simulink model "sampleModel69"  (Simulink 9.1)
settings: Solver=VariableStepAuto  StartTime=0.0  StopTime=10.0  RelTol=1e-3
undefined symbols (not defined in the file): DiscIntNeverNeededParam, Newton, Raphson
libraries: simulink x28
settings Model: SuppressorTable="22 serialization::archive 11 0 6 0 0 1 8 0 0 0 0 6 0 0 1 0 21 sampleModel69/cfblk24 0 6 0 0 2 8 0 0 0 0 6 41 Simulink:DataType:WarningOverFlowDetected 0 0 0 6 0  0  0 0 0 0 8 20160523 0 0 0 10 57 55 0 1 40 SimulinkFixedPoint:util:Overflowoccurred 0 0 0  0  8 20160523 0 10 57 55 0 1"  Creator=DELL  LastModifiedBy=DELL
settings DataIOCC: SaveFormat=Dataset
settings OptimizationCC: LifeSpan=auto
settings DebuggingCC: UnderspecifiedInitializationDetection=Simplified  MergeDetectMultiDrivingBlocksExec=error  SFUnexpectedBacktrackingDiag=error  SFNoUnconditionalDefaultTransitionDiag=error  SFExecutionAtInitializationDiag=warning
settings HardwareCC: ProdBitPerPointer=64  ProdBitPerSizeT=64  ProdBitPerPtrDiffT=64  ProdLargestAtomicFloat=Float  ProdIntDivRoundTo=Zero  ProdEndianess=LittleEndian  ProdWordSize=64  ProdHWDeviceType=Intel->x86-64 (Windows64)
settings ModelReferenceCC: PropagateSignalLabelsOutOfModel=on
settings CodeAppCC: StateflowObjectComments=off
settings GRTTargetCC: TargetLangStandard=C99 (ISO)  CombineOutputUpdateFcns=on  GRTInterface=off
settings ConfigComp: CovMetricSettings=dwe  CovHtmlReporting=off  CovSaveCumulativeToWorkspaceVar=off  CovSaveSingleToWorkspaceVar=off  CovExternalEMLEnable=on

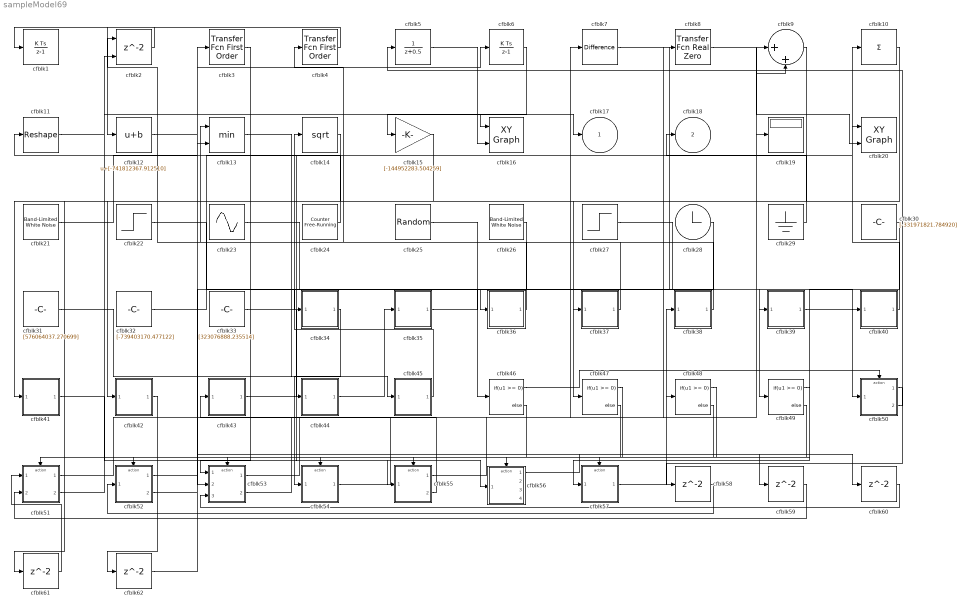
== system sampleModel69 ==
  cfblk1 : DiscreteIntegrator  ICPrevOutput=DiscIntNeverNeededParam  ICPrevScaledInput=DiscIntNeverNeededParam
  cfblk10 : Sum  Inputs=+
  cfblk11 : Reshape
  cfblk12 : Bias  Bias=[-741812367.912510]
  cfblk13 : MinMax  Inputs=2
  cfblk14 : Sqrt  SaturateOnIntegerOverflow=on
  cfblk15 : Gain  Gain=[-144952283.504259]
  cfblk16 : simulink/Sinks/XY Graph  xmin=-1  xmax=1  ymin=-1  ymax=1  st=-1
  cfblk19 : Display
  cfblk2 : Delay  ShowEnablePort=on  SampleTime=1
      settings: InputPortMap=u0,e6
  cfblk20 : simulink/Sinks/XY Graph  xmin=-1  xmax=1  ymin=-1  ymax=1  st=-1
  cfblk21 : simulink/Sources/Band-Limited White Noise  Cov=[6037447037.937979]  Ts=0.1  seed=[876082566.000000]
  cfblk22 : Step  Time=[11.000000]  Before=[-275297189.840630]  After=[-539641405.441389]  SampleTime=0
  cfblk23 : Sin  Amplitude=[-719520156.882693]  Bias=[435795628.391906]  SampleTime=0
  cfblk24 : simulink/Sources/Counter Free-Running  NumBits=[17.000000]  tsamp=-1
  cfblk25 : RandomNumber  Mean=[13472.399108]  Variance=[10146.259517]  Seed=[945900155.000000]  SampleTime=0.1
  cfblk26 : simulink/Sources/Band-Limited White Noise  Cov=[3648562607.707092]  Ts=0.1  seed=[6350696125.000000]
  cfblk27 : Step  Time=[48.000000]  Before=[68635987.034339]  After=[-934709305.033642]  SampleTime=0
  cfblk28 : Clock
  cfblk29 : Ground
  cfblk3 : simulink/Discrete/Transfer Fcn First Order  PoleZ=0.95  ICPrevOutput=0.0  DoSatur=off
      settings: SourceProductName=Simulink
  cfblk30 : Constant  Value=[-331971821.784920]  SampleTime=1
  cfblk31 : Constant  Value=[576064037.270699]  SampleTime=1
  cfblk32 : Constant  Value=[-739403170.477122]  SampleTime=1
  cfblk33 : Constant  Value=[323076888.235514]  SampleTime=1
  cfblk34 : Subsystem
  cfblk35 : Subsystem
  cfblk36 : Subsystem
  cfblk37 : Subsystem
  cfblk38 : Subsystem
  cfblk39 : Subsystem
  cfblk4 : simulink/Discrete/Transfer Fcn First Order  PoleZ=0.95  ICPrevOutput=0.0  DoSatur=off
      settings: SourceProductName=Simulink
  cfblk40 : Subsystem
  cfblk41 : Subsystem
  cfblk42 : Subsystem
  cfblk43 : Subsystem
  cfblk44 : Subsystem
  cfblk45 : Subsystem
  cfblk{46..49} (4 alike) : If  IfExpression=u1 >= 0  SampleTime=1
  cfblk5 : DiscreteTransferFcn  SampleTime=1
  cfblk50 : Subsystem  TreatAsAtomicUnit=on
  cfblk51 : Subsystem  TreatAsAtomicUnit=on
  cfblk52 : Subsystem  TreatAsAtomicUnit=on
  cfblk53 : Subsystem  TreatAsAtomicUnit=on
  cfblk54 : Subsystem  TreatAsAtomicUnit=on
  cfblk55 : Subsystem  TreatAsAtomicUnit=on
  cfblk56 : Subsystem  TreatAsAtomicUnit=on
  cfblk57 : Subsystem  TreatAsAtomicUnit=on
  cfblk{58..62} (5 alike) : Delay  SampleTime=1
  cfblk6 : DiscreteIntegrator  ICPrevOutput=DiscIntNeverNeededParam  ICPrevScaledInput=DiscIntNeverNeededParam
  cfblk7 : simulink/Discrete/Difference  ICPrevInput=0.0  OutMin=[]  OutMax=[]  OutDataTypeStr=Inherit: Inherit via back propagation  OutDataType=fixdt(1, 16)  OutScaling=2^-10  DoSatur=off
  cfblk8 : simulink/Discrete/Transfer Fcn Real Zero  ZeroZ=0.75  ICPrevInput=0.0  DoSatur=off
      settings: SourceProductName=Simulink  SourceProductBaseCode=SL
  cfblk9 : Sum  Inputs=|++
  cfblk17 : Outport
  cfblk18 : Outport  Port=2
  wires:
  cfblk34/1(cfblk2) -> cfblk54/1(cfblk1)
  cfblk23/1 -> cfblk47/1
  cfblk45/1(cfblk2) -> cfblk14/1
  cfblk22/1 -> cfblk36/1(cfblk1)
  cfblk9/1 -> cfblk41/1(cfblk1)
  cfblk13/1 -> cfblk45/1(cfblk1)
  cfblk32/1 -> cfblk10/1
  cfblk27/1 -> cfblk49/1
  cfblk7/1 -> cfblk39/1(cfblk1)
  cfblk14/1 -> cfblk42/1(cfblk1)
  cfblk30/1 -> cfblk57/1(cfblk1)
  cfblk38/1(cfblk2) -> cfblk13/1
  cfblk57/1(cfblk2) -> cfblk38/1(cfblk1)
  cfblk54/1(cfblk2) -> cfblk7/1
  cfblk24/1 -> cfblk11/1
  cfblk53/1(cfblk2) -> cfblk19/1
  cfblk40/1(cfblk2) -> cfblk20/1
  cfblk37/1(cfblk2) -> cfblk4/1
  cfblk4/1 -> cfblk12/1
  cfblk39/1(cfblk2) -> cfblk50/1(cfblk1)
  cfblk50/2(cfblk13) -> cfblk5/1
  cfblk12/1 -> cfblk16/1
  cfblk53/2(cfblk11) -> cfblk48/1
  cfblk51/1(cfblk2) -> cfblk9/1
  cfblk36/1(cfblk2) -> cfblk2/1
  cfblk3/1 -> cfblk53/1(cfblk1)
  cfblk33/1 -> cfblk55/1(cfblk1)
  cfblk2/1 -> cfblk1/1
  cfblk52/2(cfblk16) -> cfblk6/1
  cfblk8/1 -> cfblk20/2
  cfblk21/1 -> cfblk3/1
  cfblk55/1(cfblk2) -> cfblk8/1
  cfblk25/1 -> cfblk46/1
  cfblk43/1(cfblk2) -> cfblk9/2
  cfblk5/1 -> cfblk16/2
  cfblk29/1 -> cfblk18/1
  cfblk44/1(cfblk2) -> cfblk35/1(cfblk1)
  cfblk41/1(cfblk2) -> cfblk56/1(cfblk1)
  cfblk55/2(cfblk12) -> cfblk43/1(cfblk1)
  cfblk51/2(cfblk7) -> cfblk2/2
  cfblk28/1 -> cfblk34/1(cfblk1)
  cfblk10/1 -> cfblk37/1(cfblk1)
  cfblk35/1(cfblk2) -> cfblk40/1(cfblk1)
  cfblk31/1 -> cfblk44/1(cfblk1)
  cfblk26/1 -> cfblk53/2(cfblk9)
  cfblk11/1 -> cfblk17/1
  cfblk6/1 -> cfblk15/1
  cfblk46/1 -> cfblk50/Action
  cfblk46/2 -> cfblk51/Action
  cfblk47/1 -> cfblk52/Action
  cfblk47/2 -> cfblk53/Action
  cfblk48/1 -> cfblk54/Action
  cfblk48/2 -> cfblk55/Action
  cfblk49/1 -> cfblk56/Action
  cfblk49/2 -> cfblk57/Action
  cfblk50/1(cfblk2) -> cfblk58/1
  cfblk58/1 -> cfblk52/1(cfblk1)
  cfblk52/1(cfblk2) -> cfblk59/1
  cfblk59/1 -> cfblk51/2(cfblk6)
  cfblk56/1(cfblk2) -> cfblk60/1
  cfblk60/1 -> cfblk53/3(cfblk10)
  cfblk15/1 -> cfblk61/1
  cfblk61/1 -> cfblk51/1(cfblk1)
  cfblk42/1(cfblk2) -> cfblk62/1
  cfblk62/1 -> cfblk13/2

== system sampleModel69/cfblk34 ==
  cfblk1 : Inport
  cfblk2 : Outport
  wires:
  cfblk1/1 -> cfblk2/1

== system sampleModel69/cfblk35 ==
  cfblk1 : Inport
  cfblk2 : Outport
  wires:
  cfblk1/1 -> cfblk2/1

== system sampleModel69/cfblk36 ==
  cfblk1 : Inport
  cfblk2 : Outport
  wires:
  cfblk1/1 -> cfblk2/1

== system sampleModel69/cfblk37 ==
  cfblk1 : Inport
  cfblk2 : Outport
  wires:
  cfblk1/1 -> cfblk2/1

== system sampleModel69/cfblk38 ==
  cfblk1 : Inport
  cfblk2 : Outport
  wires:
  cfblk1/1 -> cfblk2/1

== system sampleModel69/cfblk39 ==
  cfblk1 : Inport
  cfblk2 : Outport
  wires:
  cfblk1/1 -> cfblk2/1

== system sampleModel69/cfblk40 ==
  cfblk1 : Inport
  cfblk2 : Outport
  wires:
  cfblk1/1 -> cfblk2/1

== system sampleModel69/cfblk41 ==
  cfblk1 : Inport
  cfblk2 : Outport
  wires:
  cfblk1/1 -> cfblk2/1

== system sampleModel69/cfblk42 ==
  cfblk1 : Inport
  cfblk2 : Outport
  wires:
  cfblk1/1 -> cfblk2/1

== system sampleModel69/cfblk43 ==
  cfblk1 : Inport
  cfblk2 : Outport
  wires:
  cfblk1/1 -> cfblk2/1

== system sampleModel69/cfblk44 ==
  cfblk1 : Inport
  cfblk2 : Outport
  wires:
  cfblk1/1 -> cfblk2/1

== system sampleModel69/cfblk45 ==
  cfblk1 : Inport
  cfblk2 : Outport
  wires:
  cfblk1/1 -> cfblk2/1

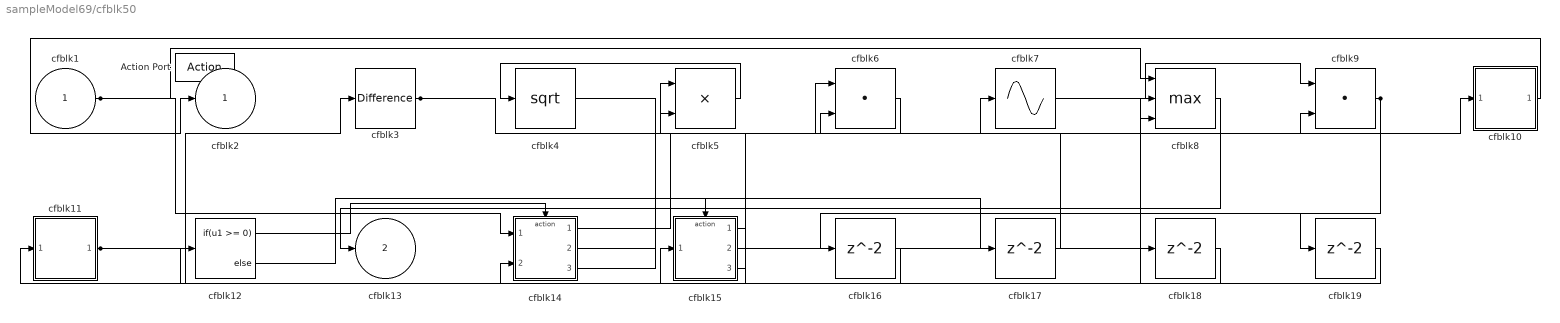
== system sampleModel69/cfblk50 ==
  cfblk1 : Inport
  Action Port : ActionPort  ActionType=then
  cfblk10 : Subsystem
  cfblk11 : Subsystem
  cfblk12 : If  IfExpression=u1 >= 0  SampleTime=1
  cfblk14 : Subsystem  TreatAsAtomicUnit=on
  cfblk15 : Subsystem  TreatAsAtomicUnit=on
  cfblk{16..19} (4 alike) : Delay
  cfblk3 : simulink/Discrete/Difference  ICPrevInput=0.0  OutMin=[]  OutMax=[]  OutDataTypeStr=Inherit: Inherit via back propagation  OutDataType=fixdt(1, 16)  OutScaling=2^-10  DoSatur=off
  cfblk4 : Sqrt  SaturateOnIntegerOverflow=on
  cfblk5 : Product  Inputs=**
  cfblk6 : DotProduct  InputSameDT=on  OutDataTypeStr=Inherit: Inherit via internal rule
  cfblk7 : Sin  TimeSource=Use external signal  SampleTime=0
  cfblk8 : MinMax  Function=max  Inputs=3
  cfblk9 : DotProduct  InputSameDT=on  OutDataTypeStr=Inherit: Inherit via internal rule
  cfblk2 : Outport
  cfblk13 : Outport  Port=2
  wires:
  cfblk8/1 -> cfblk13/1
  cfblk11/1(cfblk2) -> cfblk3/1, cfblk18/1
  cfblk5/1 -> cfblk4/1
  cfblk6/1 -> cfblk5/1
  cfblk15/1(cfblk2) -> cfblk11/1(cfblk1)
  cfblk14/1(cfblk2) -> cfblk10/1(cfblk1)
  cfblk3/1 -> cfblk6/2, cfblk8/3
  cfblk7/1 -> cfblk9/1
  cfblk1/1 -> cfblk8/1, cfblk14/1(cfblk1)
  cfblk9/1 -> cfblk16/1, cfblk19/1
  cfblk15/2(cfblk12) -> cfblk8/2
  cfblk14/2(cfblk8) -> cfblk7/1
  cfblk10/1(cfblk2) -> cfblk2/1
  cfblk15/3(cfblk13) -> cfblk5/2
  cfblk14/3(cfblk9) -> cfblk9/2
  cfblk12/1 -> cfblk14/Action
  cfblk12/2 -> cfblk15/Action
  cfblk16/1 -> cfblk15/1(cfblk1)
  cfblk4/1 -> cfblk17/1
  cfblk17/1 -> cfblk6/1
  cfblk18/1 -> cfblk12/1
  cfblk19/1 -> cfblk14/2(cfblk7)

== system sampleModel69/cfblk51 ==
  cfblk1 : Inport
  cfblk6 : Inport  Port=2
  Action Port : ActionPort  ActionType=else
  cfblk3 : DiscreteStateSpace  SampleTime=-1
  cfblk4 : simulink/Discrete/Transfer Fcn Real Zero  ZeroZ=0.75  ICPrevInput=0.0  DoSatur=off
      settings: SourceProductName=Simulink  SourceProductBaseCode=SL
  cfblk5 : Subsystem
  cfblk2 : Outport
  cfblk7 : Outport  Port=2
  wires:
  cfblk6/1 -> cfblk4/1
  cfblk1/1 -> cfblk5/1(cfblk1)
  cfblk4/1 -> cfblk7/1
  cfblk5/1(cfblk2) -> cfblk3/1
  cfblk3/1 -> cfblk2/1

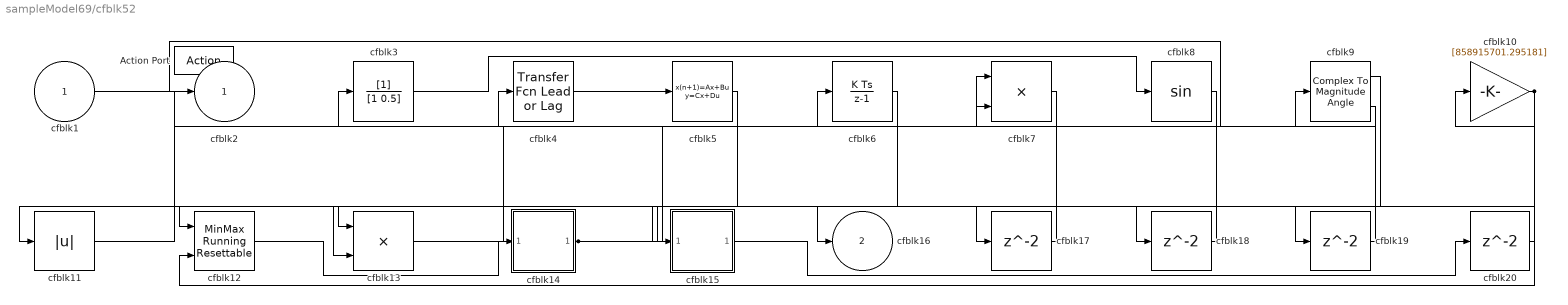
== system sampleModel69/cfblk52 ==
  cfblk1 : Inport
  Action Port : ActionPort  ActionType=then
  cfblk10 : Gain  Gain=[858915701.295181]
  cfblk11 : Abs
  cfblk12 : simulink/Math Operations/MinMax Running Resettable  Function=min  vinit=0.0
  cfblk13 : Product  Inputs=**
  cfblk14 : Subsystem
  cfblk15 : Subsystem
  cfblk{17..20} (4 alike) : Delay
  cfblk3 : DiscreteFilter
  cfblk4 : simulink/Discrete/Transfer Fcn Lead or Lag  PoleZ=0.95  ZeroZ=0.75  ICPrevOutput=0.0  ICPrevInput=0.0  DoSatur=off
      settings: SourceProductName=Simulink  SourceProductBaseCode=SL
  cfblk5 : DiscreteStateSpace  SampleTime=-1
  cfblk6 : DiscreteIntegrator  SampleTime=-1  ICPrevOutput=DiscIntNeverNeededParam  ICPrevScaledInput=DiscIntNeverNeededParam
  cfblk7 : Product  Inputs=**
  cfblk8 : Trigonometry
  cfblk9 : ComplexToMagnitudeAngle
  cfblk2 : Outport
  cfblk16 : Outport  Port=2
  wires:
  cfblk14/1(cfblk2) -> cfblk6/1, cfblk19/1
  cfblk3/1 -> cfblk8/1
  cfblk9/2 -> cfblk2/1
  cfblk4/1 -> cfblk5/1
  cfblk13/1 -> cfblk9/1
  cfblk5/1 -> cfblk12/1
  cfblk1/1 -> cfblk7/1
  cfblk7/1 -> cfblk13/2
  cfblk11/1 -> cfblk7/2
  cfblk10/1 -> cfblk12/2, cfblk16/1, cfblk15/1(cfblk1)
  cfblk12/1 -> cfblk14/1(cfblk1)
  cfblk6/1 -> cfblk11/1
  cfblk9/1 -> cfblk17/1
  cfblk17/1 -> cfblk13/1
  cfblk8/1 -> cfblk18/1
  cfblk18/1 -> cfblk3/1
  cfblk19/1 -> cfblk4/1
  cfblk15/1(cfblk2) -> cfblk20/1
  cfblk20/1 -> cfblk10/1

== system sampleModel69/cfblk53 ==
  cfblk1 : Inport
  cfblk9 : Inport  Port=2
  cfblk10 : Inport  Port=3
  Action Port : ActionPort  ActionType=else
  cfblk3 : simulink/Discrete/Difference  ICPrevInput=0.0  OutMin=[]  OutMax=[]  OutDataTypeStr=Inherit: Inherit via back propagation  OutDataType=fixdt(1, 16)  OutScaling=2^-10  DoSatur=off
  cfblk4 : DiscreteFilter
  cfblk5 : simulink/Math Operations/Slider Gain  gain=1  low=0  high=2
  cfblk6 : Sum  Inputs=+
  cfblk7 : Math  Operator=10^u  SaturateOnIntegerOverflow=on
  cfblk8 : Subsystem
  cfblk2 : Outport
  cfblk11 : Outport  Port=2
  wires:
  cfblk10/1 -> cfblk11/1
  cfblk3/1 -> cfblk7/1
  cfblk4/1 -> cfblk2/1
  cfblk9/1 -> cfblk6/1
  cfblk5/1 -> cfblk4/1
  cfblk1/1 -> cfblk3/1
  cfblk6/1 -> cfblk8/1(cfblk1)
  cfblk8/1(cfblk2) -> cfblk5/1

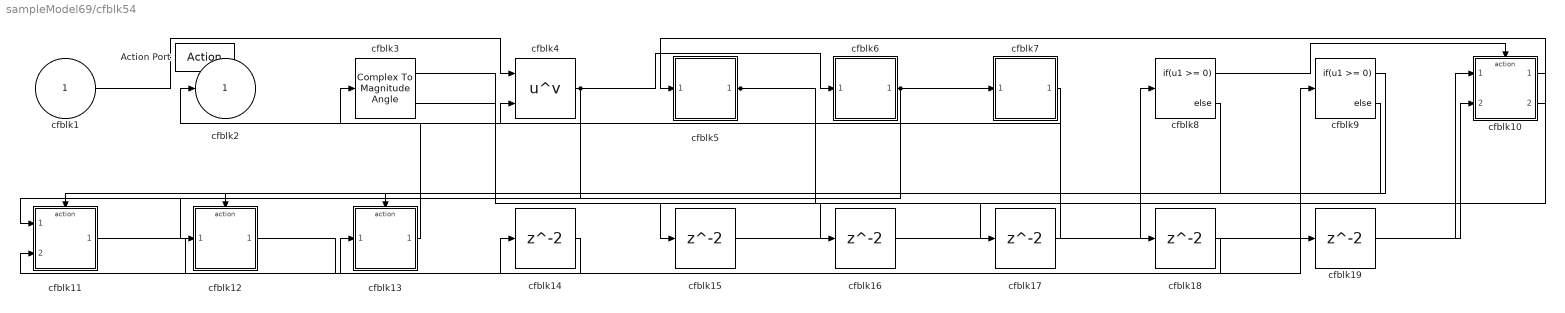
== system sampleModel69/cfblk54 ==
  cfblk1 : Inport
  Action Port : ActionPort  ActionType=then
  cfblk10 : Subsystem  TreatAsAtomicUnit=on
  cfblk11 : Subsystem  TreatAsAtomicUnit=on
  cfblk12 : Subsystem  TreatAsAtomicUnit=on
  cfblk13 : Subsystem  TreatAsAtomicUnit=on
  cfblk{14..19} (6 alike) : Delay
  cfblk3 : ComplexToMagnitudeAngle
  cfblk4 : Math  Operator=pow  SaturateOnIntegerOverflow=on
  cfblk5 : Subsystem
  cfblk6 : Subsystem
  cfblk7 : Subsystem
  cfblk8 : If  IfExpression=u1 >= 0  SampleTime=1
  cfblk9 : If  IfExpression=u1 >= 0  SampleTime=1
  cfblk2 : Outport
  wires:
  cfblk4/1 -> cfblk11/1(cfblk1), cfblk6/1(cfblk1)
  cfblk11/1(cfblk2) -> cfblk9/1
  cfblk13/1(cfblk2) -> cfblk3/1
  cfblk6/1(cfblk2) -> cfblk7/1(cfblk1), cfblk12/1(cfblk1)
  cfblk10/2(cfblk16) -> cfblk5/1(cfblk1)
  cfblk1/1 -> cfblk4/1
  cfblk5/1(cfblk2) -> cfblk17/1, cfblk18/1
  cfblk7/1(cfblk2) -> cfblk2/1
  cfblk8/1 -> cfblk10/Action
  cfblk8/2 -> cfblk11/Action
  cfblk9/1 -> cfblk12/Action
  cfblk9/2 -> cfblk13/Action
  cfblk12/1(cfblk2) -> cfblk14/1
  cfblk14/1 -> cfblk11/2(cfblk11)
  cfblk3/1 -> cfblk15/1
  cfblk15/1 -> cfblk10/1(cfblk1)
  cfblk10/1(cfblk2) -> cfblk16/1
  cfblk16/1 -> cfblk8/1
  cfblk17/1 -> cfblk4/2
  cfblk18/1 -> cfblk13/1(cfblk1)
  cfblk3/2 -> cfblk19/1
  cfblk19/1 -> cfblk10/2(cfblk15)

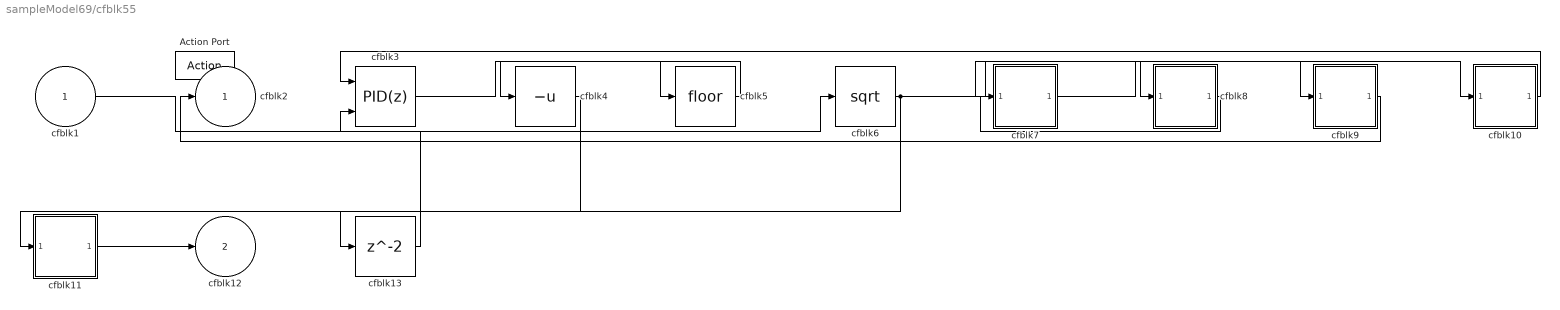
== system sampleModel69/cfblk55 ==
  cfblk1 : Inport
  Action Port : ActionPort  ActionType=else
  cfblk10 : Subsystem
  cfblk11 : Subsystem
  cfblk13 : Delay
  cfblk3 : simulink/Continuous/PID Controller (2DOF)  Controller=PID  TimeDomain=Discrete-time  SampleTime=-1  IntegratorMethod=Forward Euler  FilterMethod=Forward Euler  Form=Parallel  UseFilter=on  ControllerParametersSource=internal  P=1  I=1  D=0  N=100  b=1  c=1  InitialConditionSource=internal  InitialConditionForIntegrator=0  InitialConditionForFilter=0  ExternalReset=none  LimitOutput=off  UpperSaturationLimit=inf  LowerSaturationLimit=-inf  LinearizeAsGain=off  AntiWindupMode=none  Kb=1  TrackingMode=off  Kt=1  PParamMin=[]  PParamMax=[]  IParamMin=[]  IParamMax=[]  DParamMin=[]  DParamMax=[]  NParamMin=[]  NParamMax=[]  bParamMin=[]  bParamMax=[]  cParamMin=[]  cParamMax=[]  KbParamMin=[]  KbParamMax=[]  KtParamMin=[]  KtParamMax=[]  POutMin=[]  POutMax=[]  IOutMin=[]  IOutMax=[]  DOutMin=[]  DOutMax=[]  NOutMin=[]  NOutMax=[]  bOutMin=[]  bOutMax=[]  cOutMin=[]  cOutMax=[]  KbOutMin=[]  KbOutMax=[]  KtOutMin=[]  KtOutMax=[]  IntegratorOutMin=[]  IntegratorOutMax=[]  FilterOutMin=[]  FilterOutMax=[]  SumOutMin=[]  SumOutMax=[]  Sum1OutMin=[]  Sum1OutMax=[]  Sum2OutMin=[]  Sum2OutMax=[]  Sum3OutMin=[]  Sum3OutMax=[]  SumI1OutMin=[]  SumI1OutMax=[]  SumI2OutMin=[]  SumI2OutMax=[]  SumI3OutMin=[]  SumI3OutMax=[]  SumDOutMin=[]  SumDOutMax=[]  SaturationOutMin=[]  SaturationOutMax=[]  IntegratorContinuousStateAttributes=''  IntegratorStateMustResolveToSignalObject=off  IntegratorRTWStateStorageClass=Auto  FilterContinuousStateAttributes=''  FilterStateMustResolveToSignalObject=off  FilterRTWStateStorageClass=Auto  DifferentiatorICPrevScaledInput=0  DifferentiatorOutMin=[]  DifferentiatorOutMax=[]  FilterDiffOutCoefMin=[]  FilterDiffOutCoefMax=[]  SumDenOutMin=[]  SumDenOutMax=[]  SumNumOutMin=[]  SumNumOutMax=[]  ReciprocalOutMin=[]  ReciprocalOutMax=[]  DivideOutMin=[]  DivideOutMax=[]  TunerSelectOption=Transfer Function Based (PID Tuner App)
  cfblk4 : UnaryMinus
  cfblk5 : Rounding
  cfblk6 : Sqrt  SaturateOnIntegerOverflow=on
  cfblk7 : Subsystem
  cfblk8 : Subsystem
  cfblk9 : Subsystem
  cfblk2 : Outport
  cfblk12 : Outport  Port=2
  wires:
  cfblk6/1 -> cfblk8/1(cfblk1), cfblk11/1(cfblk1), cfblk10/1(cfblk1)
  cfblk8/1(cfblk2) -> cfblk7/1(cfblk1)
  cfblk10/1(cfblk2) -> cfblk3/1
  cfblk5/1 -> cfblk4/1
  cfblk9/1(cfblk2) -> cfblk2/1
  cfblk7/1(cfblk2) -> cfblk9/1(cfblk1)
  cfblk3/1 -> cfblk5/1
  cfblk1/1 -> cfblk6/1
  cfblk11/1(cfblk2) -> cfblk12/1
  cfblk4/1 -> cfblk13/1
  cfblk13/1 -> cfblk3/2

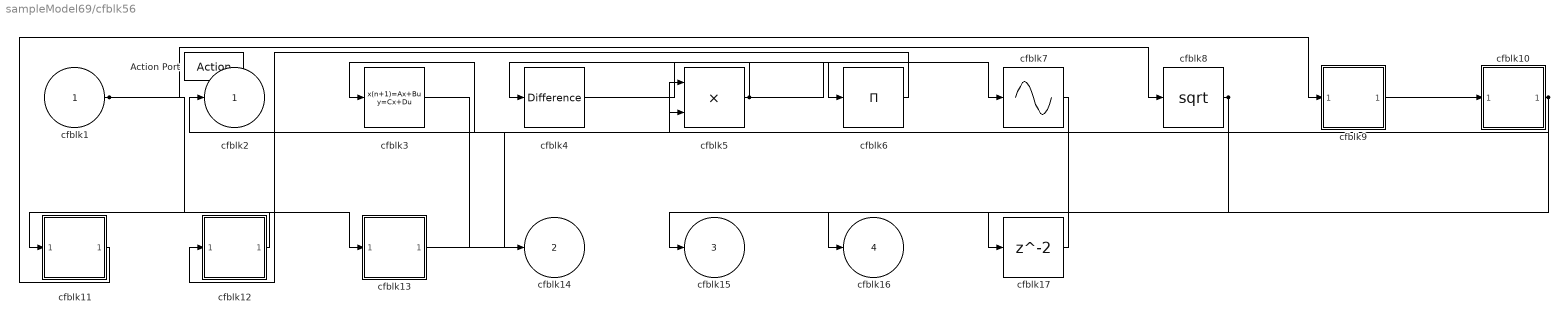
== system sampleModel69/cfblk56 ==
  cfblk1 : Inport
  Action Port : ActionPort  ActionType=then
  cfblk10 : Subsystem
  cfblk11 : Subsystem
  cfblk12 : Subsystem
  cfblk13 : Subsystem
  cfblk17 : Delay
  cfblk3 : DiscreteStateSpace  SampleTime=-1
  cfblk4 : simulink/Discrete/Difference  ICPrevInput=0.0  OutMin=[]  OutMax=[]  OutDataTypeStr=Inherit: Inherit via back propagation  OutDataType=fixdt(1, 16)  OutScaling=2^-10  DoSatur=off
  cfblk5 : Product
  cfblk6 : Product  Inputs=*
  cfblk7 : Sin  TimeSource=Use external signal  SampleTime=0
  cfblk8 : Sqrt  SaturateOnIntegerOverflow=on
  cfblk9 : Subsystem
  cfblk2 : Outport
  cfblk14 : Outport  Port=2
  cfblk15 : Outport  Port=3
  cfblk16 : Outport  Port=4
  wires:
  cfblk3/1 -> cfblk14/1
  cfblk1/1 -> cfblk8/1, cfblk13/1(cfblk1)
  cfblk10/1(cfblk2) -> cfblk3/1, cfblk17/1
  cfblk8/1 -> cfblk16/1, cfblk2/1
  cfblk7/1 -> cfblk15/1
  cfblk12/1(cfblk2) -> cfblk11/1(cfblk1)
  cfblk4/1 -> cfblk6/1
  cfblk9/1(cfblk2) -> cfblk10/1(cfblk1)
  cfblk5/1 -> cfblk4/1, cfblk7/1
  cfblk6/1 -> cfblk12/1(cfblk1)
  cfblk13/1(cfblk2) -> cfblk5/1
  cfblk11/1(cfblk2) -> cfblk9/1(cfblk1)
  cfblk17/1 -> cfblk5/2

== system sampleModel69/cfblk57 ==
  cfblk1 : Inport
  Action Port : ActionPort  ActionType=else
  cfblk10 : Subsystem
  cfblk3 : Rounding
  cfblk4 : Product  Inputs=**
  cfblk5 : simulink/Math Operations/Slider Gain  gain=1  low=0  high=2
  cfblk6 : Constant  Value=[996348552.197268]  SampleTime=1
  cfblk7 : Constant  Value=[896739633.178323]  SampleTime=1
  cfblk8 : Subsystem
  cfblk9 : Subsystem
  cfblk2 : Outport
  wires:
  cfblk9/1(cfblk2) -> cfblk3/1
  cfblk8/1(cfblk2) -> cfblk10/1(cfblk1)
  cfblk3/1 -> cfblk2/1
  cfblk10/1(cfblk2) -> cfblk5/1
  cfblk6/1 -> cfblk4/1
  cfblk7/1 -> cfblk8/1(cfblk1)
  cfblk4/1 -> cfblk9/1(cfblk1)
  cfblk5/1 -> cfblk4/2

== system sampleModel69/cfblk50/cfblk10 ==
  cfblk1 : Inport
  cfblk2 : Outport
  wires:
  cfblk1/1 -> cfblk2/1

== system sampleModel69/cfblk50/cfblk11 ==
  cfblk1 : Inport
  cfblk2 : Outport
  wires:
  cfblk1/1 -> cfblk2/1

== system sampleModel69/cfblk50/cfblk14 ==
  cfblk1 : Inport
  cfblk7 : Inport  Port=2
  Action Port : ActionPort  ActionType=then
  cfblk10 : Delay
  cfblk3 : Reshape
  cfblk4 : Subsystem
  cfblk5 : Subsystem
  cfblk6 : Subsystem
  cfblk2 : Outport
  cfblk8 : Outport  Port=2
  cfblk9 : Outport  Port=3
  wires:
  cfblk5/1(cfblk2) -> cfblk4/1(cfblk1)
  cfblk4/1(cfblk2) -> cfblk8/1, cfblk10/1
  cfblk3/1 -> cfblk5/1(cfblk1)
  cfblk6/1(cfblk2) -> cfblk9/1
  cfblk7/1 -> cfblk6/1(cfblk1)
  cfblk1/1 -> cfblk2/1
  cfblk10/1 -> cfblk3/1

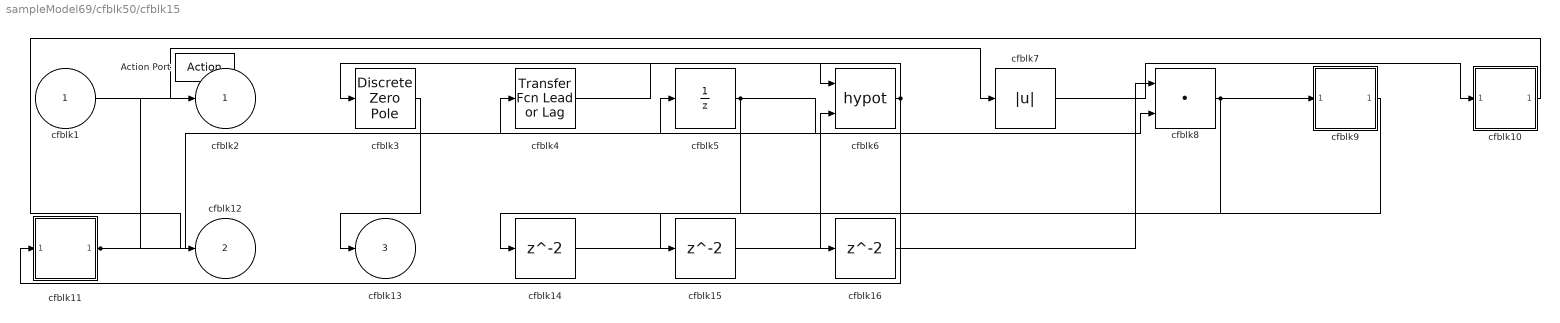
== system sampleModel69/cfblk50/cfblk15 ==
  cfblk1 : Inport
  Action Port : ActionPort  ActionType=else
  cfblk10 : Subsystem
  cfblk11 : Subsystem
  cfblk14 : Delay
  cfblk15 : Delay
  cfblk16 : Delay
  cfblk3 : DiscreteZeroPole  Poles=[0 0.5]  Gain=1  SampleTime=-1
  cfblk4 : simulink/Discrete/Transfer Fcn Lead or Lag  PoleZ=0.95  ZeroZ=0.75  ICPrevOutput=0.0  ICPrevInput=0.0  DoSatur=off
      settings: SourceProductName=Simulink  SourceProductBaseCode=SL
  cfblk5 : UnitDelay  SampleTime=-1
  cfblk6 : Math  Operator=hypot  SaturateOnIntegerOverflow=on
  cfblk7 : Abs
  cfblk8 : DotProduct  InputSameDT=on  OutDataTypeStr=Inherit: Inherit via internal rule
  cfblk9 : Subsystem
  cfblk2 : Outport
  cfblk12 : Outport  Port=2
  cfblk13 : Outport  Port=3
  wires:
  cfblk11/1(cfblk2) -> cfblk5/1, cfblk2/1
  cfblk6/1 -> cfblk11/1(cfblk1), cfblk3/1
  cfblk1/1 -> cfblk7/1
  cfblk4/1 -> cfblk6/1
  cfblk5/1 -> cfblk8/2, cfblk14/1
  cfblk7/1 -> cfblk10/1(cfblk1)
  cfblk8/1 -> cfblk9/1(cfblk1), cfblk16/1
  cfblk10/1(cfblk2) -> cfblk12/1
  cfblk3/1 -> cfblk13/1
  cfblk14/1 -> cfblk6/2
  cfblk9/1(cfblk2) -> cfblk15/1
  cfblk15/1 -> cfblk8/1
  cfblk16/1 -> cfblk4/1

== system sampleModel69/cfblk51/cfblk5 ==
  cfblk1 : Inport
  cfblk2 : Outport
  wires:
  cfblk1/1 -> cfblk2/1

== system sampleModel69/cfblk52/cfblk14 ==
  cfblk1 : Inport
  cfblk2 : Outport
  wires:
  cfblk1/1 -> cfblk2/1

== system sampleModel69/cfblk52/cfblk15 ==
  cfblk1 : Inport
  cfblk2 : Outport
  wires:
  cfblk1/1 -> cfblk2/1

== system sampleModel69/cfblk53/cfblk8 ==
  cfblk1 : Inport
  cfblk2 : Outport
  wires:
  cfblk1/1 -> cfblk2/1

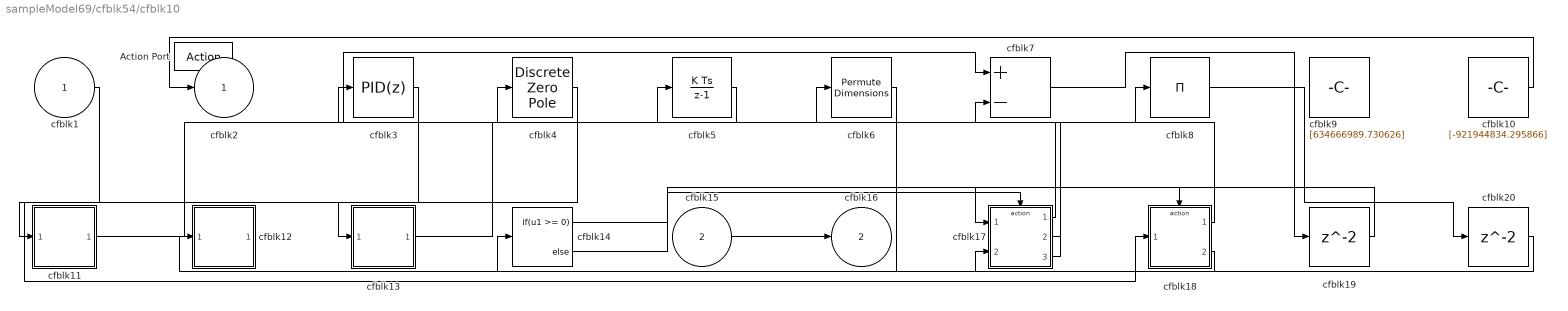
== system sampleModel69/cfblk54/cfblk10 ==
  cfblk1 : Inport
  cfblk15 : Inport  Port=2
  Action Port : ActionPort  ActionType=then
  cfblk10 : Constant  Value=[-921944834.295866]  SampleTime=1
  cfblk11 : Subsystem
  cfblk12 : Subsystem
  cfblk13 : Subsystem
  cfblk14 : If  IfExpression=u1 >= 0  SampleTime=1
  cfblk17 : Subsystem  TreatAsAtomicUnit=on
  cfblk18 : Subsystem  TreatAsAtomicUnit=on
  cfblk19 : Delay
  cfblk20 : Delay
  cfblk3 : simulink/Continuous/PID Controller  Controller=PID  TimeDomain=Discrete-time  SampleTime=-1  IntegratorMethod=Forward Euler  FilterMethod=Forward Euler  Form=Parallel  UseFilter=on  ControllerParametersSource=internal  P=1  I=1  D=0  N=100  InitialConditionSource=internal  InitialConditionForIntegrator=0  InitialConditionForFilter=0  ExternalReset=none  LimitOutput=off  UpperSaturationLimit=inf  LowerSaturationLimit=-inf  LinearizeAsGain=off  AntiWindupMode=none  Kb=1  TrackingMode=off  Kt=1  PParamMin=[]  PParamMax=[]  IParamMin=[]  IParamMax=[]  DParamMin=[]  DParamMax=[]  NParamMin=[]  NParamMax=[]  KbParamMin=[]  KbParamMax=[]  KtParamMin=[]  KtParamMax=[]  POutMin=[]  POutMax=[]  IOutMin=[]  IOutMax=[]  DOutMin=[]  DOutMax=[]  NOutMin=[]  NOutMax=[]  KbOutMin=[]  KbOutMax=[]  KtOutMin=[]  KtOutMax=[]  IntegratorOutMin=[]  IntegratorOutMax=[]  FilterOutMin=[]  FilterOutMax=[]  SumOutMin=[]  SumOutMax=[]  SumI1OutMin=[]  SumI1OutMax=[]  SumI2OutMin=[]  SumI2OutMax=[]  SumI3OutMin=[]  SumI3OutMax=[]  SumDOutMin=[]  SumDOutMax=[]  SaturationOutMin=[]  SaturationOutMax=[]  IntegratorContinuousStateAttributes=''  IntegratorStateMustResolveToSignalObject=off  IntegratorRTWStateStorageClass=Auto  FilterContinuousStateAttributes=''  FilterStateMustResolveToSignalObject=off  FilterRTWStateStorageClass=Auto  DifferentiatorICPrevScaledInput=0  DifferentiatorOutMin=[]  DifferentiatorOutMax=[]  FilterDiffOutCoefMin=[]  FilterDiffOutCoefMax=[]  SumDenOutMin=[]  SumDenOutMax=[]  SumNumOutMin=[]  SumNumOutMax=[]  ReciprocalOutMin=[]  ReciprocalOutMax=[]  DivideOutMin=[]  DivideOutMax=[]  TunerSelectOption=Transfer Function Based (PID Tuner App)
  cfblk4 : DiscreteZeroPole  Poles=[0 0.5]  Gain=1  SampleTime=-1
  cfblk5 : DiscreteIntegrator  SampleTime=-1  ICPrevOutput=DiscIntNeverNeededParam  ICPrevScaledInput=DiscIntNeverNeededParam
  cfblk6 : PermuteDimensions
  cfblk7 : Sum  Inputs=+-
  cfblk8 : Product  Inputs=*
  cfblk9 : Constant  Value=[634666989.730626]  SampleTime=1
  cfblk2 : Outport
  cfblk16 : Outport  Port=2
  wires:
  cfblk3/1 -> cfblk13/1(cfblk1)
  cfblk11/1(cfblk2) -> cfblk7/1
  cfblk6/1 -> cfblk12/1(cfblk1)
  cfblk15/1 -> cfblk16/1
  cfblk1/1 -> cfblk18/1(cfblk1)
  cfblk5/1 -> cfblk4/1
  cfblk18/1(cfblk2) -> cfblk6/1
  cfblk10/1 -> cfblk2/1
  cfblk17/1(cfblk2) -> cfblk7/2
  cfblk4/1 -> cfblk11/1(cfblk1)
  cfblk13/1(cfblk2) -> cfblk8/1
  cfblk18/2(cfblk9) -> cfblk17/2(cfblk8)
  cfblk17/2(cfblk9) -> cfblk3/1
  cfblk17/3(cfblk10) -> cfblk5/1
  cfblk14/1 -> cfblk17/Action
  cfblk14/2 -> cfblk18/Action
  cfblk7/1 -> cfblk19/1
  cfblk19/1 -> cfblk17/1(cfblk1)
  cfblk8/1 -> cfblk20/1
  cfblk20/1 -> cfblk14/1

== system sampleModel69/cfblk54/cfblk11 ==
  cfblk1 : Inport
  cfblk11 : Inport  Port=2
  Action Port : ActionPort  ActionType=else
  cfblk10 : Constant  Value=[-596378645.496508]  SampleTime=1
  cfblk3 : simulink/Discrete/Transfer Fcn First Order  PoleZ=0.95  ICPrevOutput=0.0  DoSatur=off
      settings: SourceProductName=Simulink
  cfblk4 : DiscreteZeroPole  Poles=[0 0.5]  Gain=1  SampleTime=-1
  cfblk5 : Gain  Gain=[543769298.920724]
  cfblk6 : Rounding
  cfblk7 : MinMax  Function=max
  cfblk8 : Constant  Value=[-960979569.414541]  SampleTime=1
  cfblk9 : Constant  Value=[98718357.511619]  SampleTime=1
  cfblk2 : Outport
  wires:
  cfblk10/1 -> cfblk5/1
  cfblk5/1 -> cfblk6/1
  cfblk1/1 -> cfblk3/1
  cfblk3/1 -> cfblk4/1
  cfblk9/1 -> cfblk2/1
  cfblk4/1 -> cfblk7/1

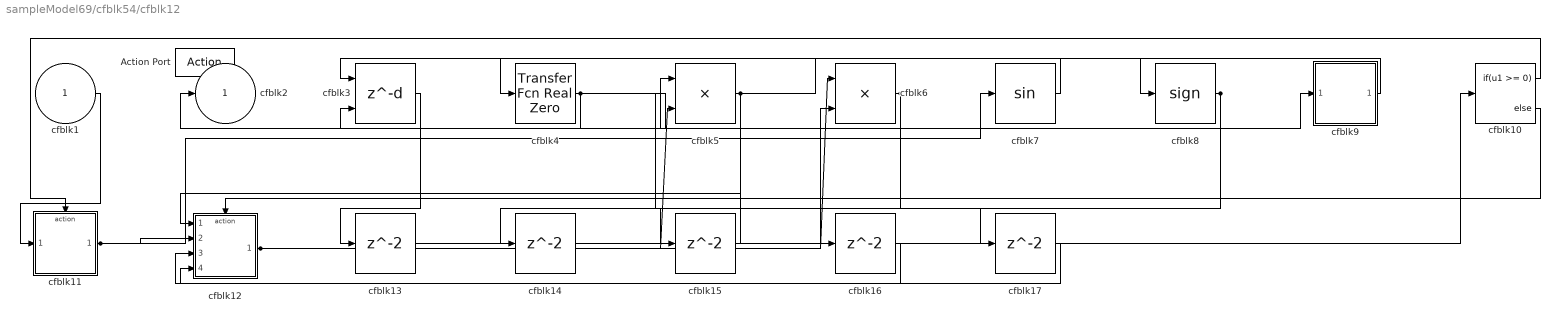
== system sampleModel69/cfblk54/cfblk12 ==
  cfblk1 : Inport
  Action Port : ActionPort  ActionType=then
  cfblk10 : If  IfExpression=u1 >= 0  SampleTime=1
  cfblk11 : Subsystem  TreatAsAtomicUnit=on
  cfblk12 : Subsystem  TreatAsAtomicUnit=on
  cfblk{13..17} (5 alike) : Delay
  cfblk3 : Delay  DelayLengthSource=Input port
      settings: InputPortMap=u0,p1
  cfblk4 : simulink/Discrete/Transfer Fcn Real Zero  ZeroZ=0.75  ICPrevInput=0.0  DoSatur=off
      settings: SourceProductName=Simulink  SourceProductBaseCode=SL
  cfblk5 : Product  Inputs=**
  cfblk6 : Product  Inputs=**
  cfblk7 : Trigonometry
  cfblk8 : Signum
  cfblk9 : Subsystem
  cfblk2 : Outport
  wires:
  cfblk9/1(cfblk2) -> cfblk3/1
  cfblk6/1 -> cfblk5/1, cfblk16/1
  cfblk11/1(cfblk2) -> cfblk7/1, cfblk12/2(cfblk8)
  cfblk7/1 -> cfblk4/1
  cfblk12/1(cfblk2) -> cfblk6/1, cfblk5/2
  cfblk8/1 -> cfblk2/1, cfblk15/1
  cfblk4/1 -> cfblk3/2, cfblk9/1(cfblk1), cfblk17/1
  cfblk5/1 -> cfblk8/1, cfblk14/1
  cfblk1/1 -> cfblk11/1(cfblk1)
  cfblk10/1 -> cfblk11/Action
  cfblk10/2 -> cfblk12/Action
  cfblk3/1 -> cfblk13/1
  cfblk13/1 -> cfblk10/1
  cfblk14/1 -> cfblk6/2
  cfblk15/1 -> cfblk12/1(cfblk1)
  cfblk16/1 -> cfblk12/3(cfblk9)
  cfblk17/1 -> cfblk12/4(cfblk10)

== system sampleModel69/cfblk54/cfblk13 ==
  cfblk1 : Inport
  Action Port : ActionPort  ActionType=else
  cfblk3 : Sum
  cfblk4 : PermuteDimensions
  cfblk5 : Product  Inputs=**
  cfblk6 : Subsystem
  cfblk7 : Subsystem
  cfblk8 : Delay
  cfblk9 : Delay
  cfblk2 : Outport
  wires:
  cfblk1/1 -> cfblk5/1
  cfblk4/1 -> cfblk7/1(cfblk1)
  cfblk3/1 -> cfblk6/1(cfblk1)
  cfblk5/1 -> cfblk3/1, cfblk3/2
  cfblk6/1(cfblk2) -> cfblk2/1, cfblk8/1
  cfblk8/1 -> cfblk5/2
  cfblk7/1(cfblk2) -> cfblk9/1
  cfblk9/1 -> cfblk4/1

== system sampleModel69/cfblk54/cfblk5 ==
  cfblk1 : Inport
  cfblk2 : Outport
  wires:
  cfblk1/1 -> cfblk2/1

== system sampleModel69/cfblk54/cfblk6 ==
  cfblk1 : Inport
  cfblk2 : Outport
  wires:
  cfblk1/1 -> cfblk2/1

== system sampleModel69/cfblk54/cfblk7 ==
  cfblk1 : Inport
  cfblk2 : Outport
  wires:
  cfblk1/1 -> cfblk2/1

== system sampleModel69/cfblk55/cfblk10 ==
  cfblk1 : Inport
  cfblk2 : Outport
  wires:
  cfblk1/1 -> cfblk2/1

== system sampleModel69/cfblk55/cfblk11 ==
  cfblk1 : Inport
  cfblk2 : Outport
  wires:
  cfblk1/1 -> cfblk2/1

== system sampleModel69/cfblk55/cfblk7 ==
  cfblk1 : Inport
  cfblk2 : Outport
  wires:
  cfblk1/1 -> cfblk2/1

== system sampleModel69/cfblk55/cfblk8 ==
  cfblk1 : Inport
  cfblk2 : Outport
  wires:
  cfblk1/1 -> cfblk2/1

== system sampleModel69/cfblk55/cfblk9 ==
  cfblk1 : Inport
  cfblk2 : Outport
  wires:
  cfblk1/1 -> cfblk2/1

== system sampleModel69/cfblk56/cfblk10 ==
  cfblk1 : Inport
  cfblk2 : Outport
  wires:
  cfblk1/1 -> cfblk2/1

== system sampleModel69/cfblk56/cfblk11 ==
  cfblk1 : Inport
  cfblk2 : Outport
  wires:
  cfblk1/1 -> cfblk2/1

== system sampleModel69/cfblk56/cfblk12 ==
  cfblk1 : Inport
  cfblk2 : Outport
  wires:
  cfblk1/1 -> cfblk2/1

== system sampleModel69/cfblk56/cfblk13 ==
  cfblk1 : Inport
  cfblk2 : Outport
  wires:
  cfblk1/1 -> cfblk2/1

== system sampleModel69/cfblk56/cfblk9 ==
  cfblk1 : Inport
  cfblk2 : Outport
  wires:
  cfblk1/1 -> cfblk2/1

== system sampleModel69/cfblk57/cfblk10 ==
  cfblk1 : Inport
  cfblk2 : Outport
  wires:
  cfblk1/1 -> cfblk2/1

== system sampleModel69/cfblk57/cfblk8 ==
  cfblk1 : Inport
  cfblk2 : Outport
  wires:
  cfblk1/1 -> cfblk2/1

== system sampleModel69/cfblk57/cfblk9 ==
  cfblk1 : Inport
  cfblk2 : Outport
  wires:
  cfblk1/1 -> cfblk2/1

== system sampleModel69/cfblk50/cfblk14/cfblk4 ==
  cfblk1 : Inport
  cfblk2 : Outport
  wires:
  cfblk1/1 -> cfblk2/1

== system sampleModel69/cfblk50/cfblk14/cfblk5 ==
  cfblk1 : Inport
  cfblk2 : Outport
  wires:
  cfblk1/1 -> cfblk2/1

== system sampleModel69/cfblk50/cfblk14/cfblk6 ==
  cfblk1 : Inport
  cfblk2 : Outport
  wires:
  cfblk1/1 -> cfblk2/1

== system sampleModel69/cfblk50/cfblk15/cfblk10 ==
  cfblk1 : Inport
  cfblk2 : Outport
  wires:
  cfblk1/1 -> cfblk2/1

== system sampleModel69/cfblk50/cfblk15/cfblk11 ==
  cfblk1 : Inport
  cfblk2 : Outport
  wires:
  cfblk1/1 -> cfblk2/1

== system sampleModel69/cfblk50/cfblk15/cfblk9 ==
  cfblk1 : Inport
  cfblk2 : Outport
  wires:
  cfblk1/1 -> cfblk2/1

== system sampleModel69/cfblk54/cfblk10/cfblk11 ==
  cfblk1 : Inport
  cfblk2 : Outport
  wires:
  cfblk1/1 -> cfblk2/1

== system sampleModel69/cfblk54/cfblk10/cfblk12 ==
  cfblk1 : Inport
  cfblk2 : Outport
  wires:
  cfblk1/1 -> cfblk2/1

== system sampleModel69/cfblk54/cfblk10/cfblk13 ==
  cfblk1 : Inport
  cfblk2 : Outport
  wires:
  cfblk1/1 -> cfblk2/1

== system sampleModel69/cfblk54/cfblk10/cfblk17 ==
  cfblk1 : Inport
  cfblk8 : Inport  Port=2
  Action Port : ActionPort  ActionType=then
  cfblk3 : DiscreteFir
  cfblk4 : DiscreteStateSpace  SampleTime=-1
  cfblk5 : ComplexToRealImag
  cfblk6 : Sqrt  Operator=rSqrt  AlgorithmType=Newton-Raphson  SaturateOnIntegerOverflow=on
  cfblk7 : Subsystem
  cfblk2 : Outport
  cfblk9 : Outport  Port=2
  cfblk10 : Outport  Port=3
  wires:
  cfblk3/1 -> cfblk5/1
  cfblk6/1 -> cfblk2/1
  cfblk8/1 -> cfblk7/1(cfblk1)
  cfblk5/1 -> cfblk9/1
  cfblk4/1 -> cfblk6/1
  cfblk7/1(cfblk2) -> cfblk3/1
  cfblk5/2 -> cfblk4/1
  cfblk1/1 -> cfblk10/1

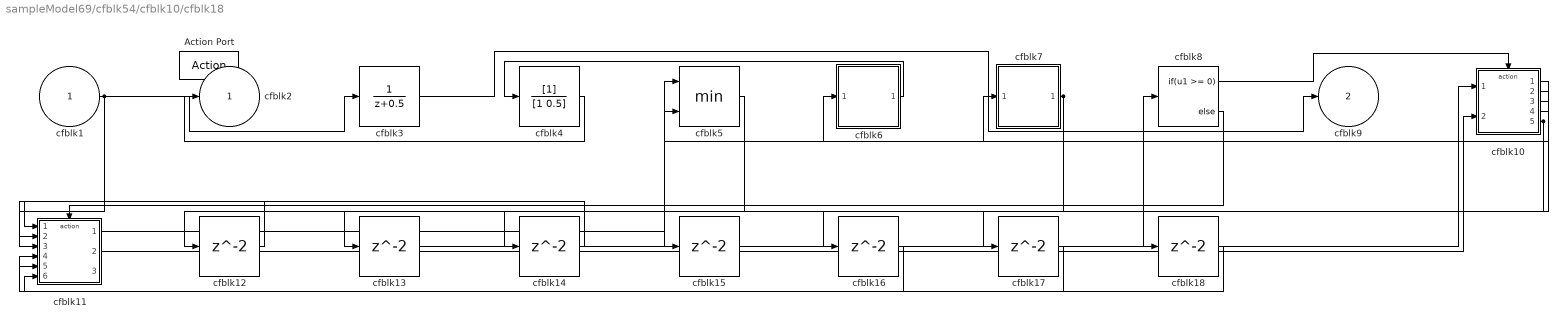
== system sampleModel69/cfblk54/cfblk10/cfblk18 ==
  cfblk1 : Inport
  Action Port : ActionPort  ActionType=else
  cfblk10 : Subsystem  TreatAsAtomicUnit=on
  cfblk11 : Subsystem  TreatAsAtomicUnit=on
  cfblk{12..18} (7 alike) : Delay
  cfblk3 : DiscreteTransferFcn
  cfblk4 : DiscreteFilter
  cfblk5 : MinMax  Inputs=2
  cfblk6 : Subsystem
  cfblk7 : Subsystem
  cfblk8 : If  IfExpression=u1 >= 0  SampleTime=1
  cfblk2 : Outport
  cfblk9 : Outport  Port=2
  wires:
  cfblk7/1(cfblk2) -> cfblk15/1, cfblk16/1
  cfblk1/1 -> cfblk3/1, cfblk11/3(cfblk11)
  cfblk6/1(cfblk2) -> cfblk4/1
  cfblk10/2(cfblk8) -> cfblk6/1(cfblk1)
  cfblk4/1 -> cfblk2/1
  cfblk3/1 -> cfblk9/1
  cfblk11/1(cfblk2) -> cfblk5/1
  cfblk10/4(cfblk10) -> cfblk7/1(cfblk1)
  cfblk10/5(cfblk11) -> cfblk5/2, cfblk17/1, cfblk18/1
  cfblk11/2(cfblk15) -> cfblk10/2(cfblk7)
  cfblk8/1 -> cfblk10/Action
  cfblk8/2 -> cfblk11/Action
  cfblk5/1 -> cfblk12/1
  cfblk12/1 -> cfblk11/1(cfblk1)
  cfblk10/1(cfblk2) -> cfblk13/1
  cfblk13/1 -> cfblk8/1
  cfblk10/3(cfblk9) -> cfblk14/1
  cfblk14/1 -> cfblk11/2(cfblk10)
  cfblk15/1 -> cfblk10/1(cfblk1)
  cfblk16/1 -> cfblk11/5(cfblk13)
  cfblk17/1 -> cfblk11/4(cfblk12)
  cfblk18/1 -> cfblk11/6(cfblk14)

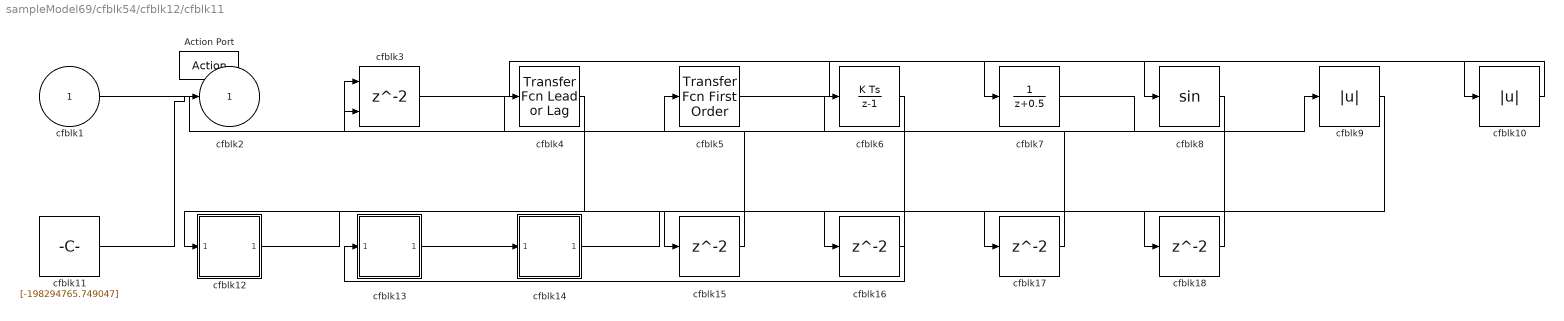
== system sampleModel69/cfblk54/cfblk12/cfblk11 ==
  cfblk1 : Inport
  Action Port : ActionPort  ActionType=then
  cfblk10 : Abs
  cfblk11 : Constant  Value=[-198294765.749047]  SampleTime=1
  cfblk12 : Subsystem
  cfblk13 : Subsystem
  cfblk14 : Subsystem
  cfblk{15..18} (4 alike) : Delay
  cfblk3 : Delay  ShowEnablePort=on
      settings: InputPortMap=u0,e6
  cfblk4 : simulink/Discrete/Transfer Fcn Lead or Lag  PoleZ=0.95  ZeroZ=0.75  ICPrevOutput=0.0  ICPrevInput=0.0  DoSatur=off
      settings: SourceProductName=Simulink  SourceProductBaseCode=SL
  cfblk5 : simulink/Discrete/Transfer Fcn First Order  PoleZ=0.95  ICPrevOutput=0.0  DoSatur=off
      settings: SourceProductName=Simulink
  cfblk6 : DiscreteIntegrator  SampleTime=-1  ICPrevOutput=DiscIntNeverNeededParam  ICPrevScaledInput=DiscIntNeverNeededParam
  cfblk7 : DiscreteTransferFcn
  cfblk8 : Trigonometry
  cfblk9 : Abs
  cfblk2 : Outport
  wires:
  cfblk3/1 -> cfblk7/1
  cfblk10/1 -> cfblk8/1
  cfblk4/1 -> cfblk12/1(cfblk1)
  cfblk6/1 -> cfblk13/1(cfblk1)
  cfblk13/1(cfblk2) -> cfblk14/1(cfblk1)
  cfblk1/1 -> cfblk3/1
  cfblk11/1 -> cfblk2/1
  cfblk7/1 -> cfblk9/1
  cfblk5/1 -> cfblk10/1
  cfblk9/1 -> cfblk15/1
  cfblk15/1 -> cfblk3/2
  cfblk12/1(cfblk2) -> cfblk16/1
  cfblk16/1 -> cfblk4/1
  cfblk8/1 -> cfblk17/1
  cfblk17/1 -> cfblk5/1
  cfblk14/1(cfblk2) -> cfblk18/1
  cfblk18/1 -> cfblk6/1

== system sampleModel69/cfblk54/cfblk12/cfblk12 ==
  cfblk1 : Inport
  cfblk8 : Inport  Port=2
  cfblk9 : Inport  Port=3
  cfblk10 : Inport  Port=4
  Action Port : ActionPort  ActionType=else
  cfblk11 : Delay
  cfblk3 : ComplexToRealImag
  cfblk4 : MinMax  Inputs=2
  cfblk5 : Sqrt  SaturateOnIntegerOverflow=on
  cfblk6 : Subsystem
  cfblk7 : Subsystem
  cfblk2 : Outport
  wires:
  cfblk1/1 -> cfblk4/1
  cfblk4/1 -> cfblk3/1
  cfblk7/1(cfblk2) -> cfblk6/1(cfblk1)
  cfblk8/1 -> cfblk5/1
  cfblk6/1(cfblk2) -> cfblk2/1
  cfblk5/1 -> cfblk7/1(cfblk1)
  cfblk3/1 -> cfblk11/1
  cfblk11/1 -> cfblk4/2

== system sampleModel69/cfblk54/cfblk12/cfblk9 ==
  cfblk1 : Inport
  cfblk2 : Outport
  wires:
  cfblk1/1 -> cfblk2/1

== system sampleModel69/cfblk54/cfblk13/cfblk6 ==
  cfblk1 : Inport
  cfblk2 : Outport
  wires:
  cfblk1/1 -> cfblk2/1

== system sampleModel69/cfblk54/cfblk13/cfblk7 ==
  cfblk1 : Inport
  cfblk2 : Outport
  wires:
  cfblk1/1 -> cfblk2/1

== system sampleModel69/cfblk54/cfblk10/cfblk17/cfblk7 ==
  cfblk1 : Inport
  cfblk2 : Outport
  wires:
  cfblk1/1 -> cfblk2/1

== system sampleModel69/cfblk54/cfblk10/cfblk18/cfblk10 ==
  cfblk1 : Inport
  cfblk7 : Inport  Port=2
  Action Port : ActionPort  ActionType=then
  cfblk3 : simulink/Discrete/Transfer Fcn Real Zero  ZeroZ=0.75  ICPrevInput=0.0  DoSatur=off
      settings: SourceProductName=Simulink  SourceProductBaseCode=SL
  cfblk4 : Product  Inputs=**
  cfblk5 : Sum  Inputs=+-
  cfblk6 : Sum  Inputs=-+
  cfblk2 : Outport
  cfblk8 : Outport  Port=2
  cfblk9 : Outport  Port=3
  cfblk10 : Outport  Port=4
  cfblk11 : Outport  Port=5
  wires:
  cfblk3/1 -> cfblk11/1
  cfblk5/1 -> cfblk2/1
  cfblk7/1 -> cfblk10/1, cfblk5/2, cfblk4/1, cfblk6/1
  cfblk4/1 -> cfblk9/1
  cfblk6/1 -> cfblk5/1, cfblk8/1
  cfblk1/1 -> cfblk3/1, cfblk4/2, cfblk6/2

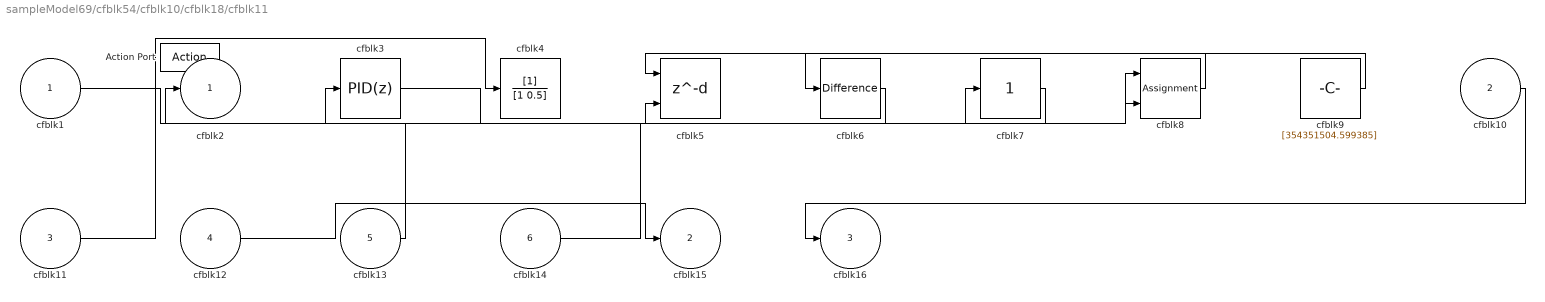
== system sampleModel69/cfblk54/cfblk10/cfblk18/cfblk11 ==
  cfblk1 : Inport
  cfblk10 : Inport  Port=2
  cfblk11 : Inport  Port=3
  cfblk12 : Inport  Port=4
  cfblk13 : Inport  Port=5
  cfblk14 : Inport  Port=6
  Action Port : ActionPort  ActionType=else
  cfblk3 : simulink/Continuous/PID Controller  Controller=PID  TimeDomain=Discrete-time  SampleTime=-1  IntegratorMethod=Forward Euler  FilterMethod=Forward Euler  Form=Parallel  UseFilter=on  ControllerParametersSource=internal  P=1  I=1  D=0  N=100  InitialConditionSource=internal  InitialConditionForIntegrator=0  InitialConditionForFilter=0  ExternalReset=none  LimitOutput=off  UpperSaturationLimit=inf  LowerSaturationLimit=-inf  LinearizeAsGain=off  AntiWindupMode=none  Kb=1  TrackingMode=off  Kt=1  PParamMin=[]  PParamMax=[]  IParamMin=[]  IParamMax=[]  DParamMin=[]  DParamMax=[]  NParamMin=[]  NParamMax=[]  KbParamMin=[]  KbParamMax=[]  KtParamMin=[]  KtParamMax=[]  POutMin=[]  POutMax=[]  IOutMin=[]  IOutMax=[]  DOutMin=[]  DOutMax=[]  NOutMin=[]  NOutMax=[]  KbOutMin=[]  KbOutMax=[]  KtOutMin=[]  KtOutMax=[]  IntegratorOutMin=[]  IntegratorOutMax=[]  FilterOutMin=[]  FilterOutMax=[]  SumOutMin=[]  SumOutMax=[]  SumI1OutMin=[]  SumI1OutMax=[]  SumI2OutMin=[]  SumI2OutMax=[]  SumI3OutMin=[]  SumI3OutMax=[]  SumDOutMin=[]  SumDOutMax=[]  SaturationOutMin=[]  SaturationOutMax=[]  IntegratorContinuousStateAttributes=''  IntegratorStateMustResolveToSignalObject=off  IntegratorRTWStateStorageClass=Auto  FilterContinuousStateAttributes=''  FilterStateMustResolveToSignalObject=off  FilterRTWStateStorageClass=Auto  DifferentiatorICPrevScaledInput=0  DifferentiatorOutMin=[]  DifferentiatorOutMax=[]  FilterDiffOutCoefMin=[]  FilterDiffOutCoefMax=[]  SumDenOutMin=[]  SumDenOutMax=[]  SumNumOutMin=[]  SumNumOutMax=[]  ReciprocalOutMin=[]  ReciprocalOutMax=[]  DivideOutMin=[]  DivideOutMax=[]  TunerSelectOption=Transfer Function Based (PID Tuner App)
  cfblk4 : DiscreteFilter
  cfblk5 : Delay  DelayLengthSource=Input port
      settings: InputPortMap=u0,p1
  cfblk6 : simulink/Discrete/Difference  ICPrevInput=0.0  OutMin=[]  OutMax=[]  OutDataTypeStr=Inherit: Inherit via back propagation  OutDataType=fixdt(1, 16)  OutScaling=2^-10  DoSatur=off
  cfblk7 : simulink/Math Operations/Slider Gain  gain=1  low=0  high=2
  cfblk8 : Assignment  DiagnosticForDimensions=Warning  IndexOptions=Index vector (dialog)  Indices=1  OutputSizes=1
  cfblk9 : Constant  Value=[354351504.599385]  SampleTime=1
  cfblk2 : Outport
  cfblk15 : Outport  Port=2
  cfblk16 : Outport  Port=3
  wires:
  cfblk10/1 -> cfblk16/1
  cfblk7/1 -> cfblk2/1
  cfblk11/1 -> cfblk4/1
  cfblk9/1 -> cfblk6/1
  cfblk12/1 -> cfblk15/1
  cfblk8/1 -> cfblk5/1
  cfblk13/1 -> cfblk3/1
  cfblk1/1 -> cfblk8/1
  cfblk14/1 -> cfblk7/1
  cfblk6/1 -> cfblk5/2
  cfblk3/1 -> cfblk8/2

== system sampleModel69/cfblk54/cfblk10/cfblk18/cfblk6 ==
  cfblk1 : Inport
  cfblk2 : Outport
  wires:
  cfblk1/1 -> cfblk2/1

== system sampleModel69/cfblk54/cfblk10/cfblk18/cfblk7 ==
  cfblk1 : Inport
  cfblk2 : Outport
  wires:
  cfblk1/1 -> cfblk2/1

== system sampleModel69/cfblk54/cfblk12/cfblk11/cfblk12 ==
  cfblk1 : Inport
  cfblk2 : Outport
  wires:
  cfblk1/1 -> cfblk2/1

== system sampleModel69/cfblk54/cfblk12/cfblk11/cfblk13 ==
  cfblk1 : Inport
  cfblk2 : Outport
  wires:
  cfblk1/1 -> cfblk2/1

== system sampleModel69/cfblk54/cfblk12/cfblk11/cfblk14 ==
  cfblk1 : Inport
  cfblk2 : Outport
  wires:
  cfblk1/1 -> cfblk2/1

== system sampleModel69/cfblk54/cfblk12/cfblk12/cfblk6 ==
  cfblk1 : Inport
  cfblk2 : Outport
  wires:
  cfblk1/1 -> cfblk2/1

== system sampleModel69/cfblk54/cfblk12/cfblk12/cfblk7 ==
  cfblk1 : Inport
  cfblk2 : Outport
  wires:
  cfblk1/1 -> cfblk2/1
